simulink model "umich_2d_walking"  (R2012b)
settings: Solver=ode3  StartTime=0.0  StopTime=inf  FixedStep=sample_time  RelTol=1e-3
values from neighbouring files (symbols this model uses):
  fcut_unwrap = 50    [init_umich_2d_walking.m]
  fcut_velocity = 100    [init_umich_2d_walking.m]
  sample_time = 1/update_freq    (= 0.001)    [init_umich_2d_walking.m]
undefined symbols (not defined in the file or in its folder): BOOM_MAX_ENCODER_TICKS, boom_mount_angle, BOOM_PITCH_CAL_VALUE_RAD, BOOM_PITCH_CAL_VALUE_TICKS, BOOM_PITCH_ENCODER_RAD_PER_TICK, BOOM_ROLL_CAL_VALUE_RAD, BOOM_ROLL_CAL_VALUE_TICKS, BOOM_ROLL_ENCODER_RAD_PER_TICK, BOOM_YAW_ENCODER_RAD_PER_TICK, control_start_time, desired_torso_pitch, DiscIntNeverNeededParam, fcut_acceleration, gd, get, h_alpha, HIP_ABS_ENCODER_RAD_PER_TICK, hip_gravity_compensation, HIP_INC_ENCODER_RAD_PER_TICK, HIP_INC_MAX_ENCODER_TICKS, HIP_MOTOR_CONSTANT, HIP_MTR_GEAR_RATIO, HIP_MTR_MAX_TORQUE, i_limit_lateral, j_motor_reflected, k_leg_spring, kd_lateral, kd_pitch, kd_sea_torque, ki_lateral, kp_lateral, kp_pitch, kp_sea_torque, lateral_torque_ramp_time, LEFT_HIP_CALIB_POS, LEFT_HIP_CALIB_VAL, LEFT_MOTOR_HIP_DIRECTION, LEG1_LEG_A_CALIB_VAL, LEG1_LEG_A_RAD_PER_CNT, LEG1_LEG_B_CALIB_VAL, LEG1_LEG_B_RAD_PER_CNT, LEG1_MOTOR_A_DIRECTION, LEG1_MOTOR_B_DIRECTION, LEG1_TRAN_A_CALIB_VAL, LEG1_TRAN_A_RAD_PER_CNT, LEG1_TRAN_B_CALIB_VAL, LEG1_TRAN_B_RAD_PER_CNT, LEG2_LEG_A_CALIB_VAL, LEG2_LEG_A_RAD_PER_CNT, LEG2_LEG_B_CALIB_VAL, LEG2_LEG_B_RAD_PER_CNT, LEG2_MOTOR_A_DIRECTION, LEG2_MOTOR_B_DIRECTION, LEG2_TRAN_A_CALIB_VAL, LEG2_TRAN_A_RAD_PER_CNT, LEG2_TRAN_B_CALIB_VAL, LEG2_TRAN_B_RAD_PER_CNT, LEG_A_CALIB_LOC, LEG_B_CALIB_LOC, LEG_MOTOR_CONSTANT ... (+23)
libraries: xpcethercatlib x160, simulink x9, dspswit3 x1
(part 3 of 3)

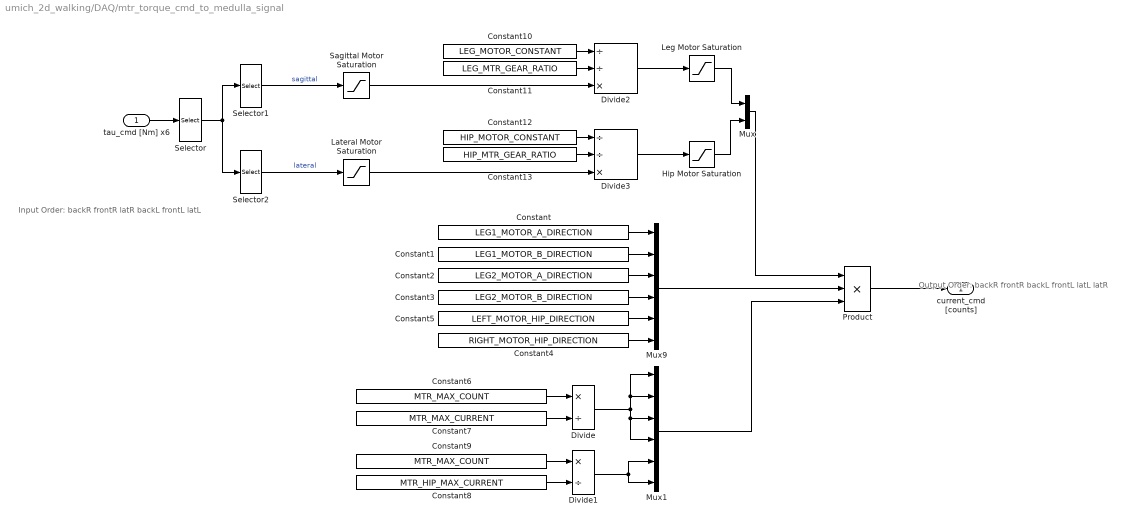
== system umich_2d_walking/DAQ/mtr_torque_cmd_to_medulla_signal ==
  note: Input Order:
      |
      | backR
      | frontR
      | latR
      | backL
      | frontL
      | latL
  note: Output Order:
      |
      | backR
      | frontR
      | backL
      | frontL
      | latL
      | latR
  tau_cmd [Nm] x6 : Inport
  " Lateral Motor Saturation" : Saturate  UpperLimit=HIP_MTR_MAX_TORQUE  LowerLimit=-HIP_MTR_MAX_TORQUE
      settings: AttributesFormatString=Top: %<UpperLimit>\nBottom: %<LowerLimit>
  " Sagittal Motor Saturation" : Saturate  UpperLimit=LEG_MTR_MAX_TORQUE  LowerLimit=-LEG_MTR_MAX_TORQUE
      settings: AttributesFormatString=Top: %<UpperLimit>\nBottom: %<LowerLimit>
  Constant : Constant  Value=LEG1_MOTOR_A_DIRECTION
  Constant1 : Constant  Value=LEG1_MOTOR_B_DIRECTION
  Constant10 : Constant  Value=LEG_MOTOR_CONSTANT
  Constant11 : Constant  Value=LEG_MTR_GEAR_RATIO
  Constant12 : Constant  Value=HIP_MOTOR_CONSTANT
  Constant13 : Constant  Value=HIP_MTR_GEAR_RATIO
  Constant2 : Constant  Value=LEG2_MOTOR_A_DIRECTION
  Constant3 : Constant  Value=LEG2_MOTOR_B_DIRECTION
  Constant4 : Constant  Value=RIGHT_MOTOR_HIP_DIRECTION
  Constant5 : Constant  Value=LEFT_MOTOR_HIP_DIRECTION
  Constant6 : Constant  Value=MTR_MAX_COUNT
  Constant7 : Constant  Value=MTR_MAX_CURRENT
  Constant8 : Constant  Value=MTR_HIP_MAX_CURRENT
  Constant9 : Constant  Value=MTR_MAX_COUNT
  Divide : Product  Inputs=*/
  Divide1 : Product  Inputs=*/
  Divide2 : Product  Inputs=//*
  Divide3 : Product  Inputs=//*
  Hip Motor Saturation : Saturate  UpperLimit=10  LowerLimit=-10
      settings: AttributesFormatString=Top: %<UpperLimit>\nBottom: %<LowerLimit>
  Leg Motor Saturation : Saturate  UpperLimit=30  LowerLimit=-30
      settings: AttributesFormatString=Top: %<UpperLimit>\nBottom: %<LowerLimit>
  Mux : Mux  Inputs=2
  Mux1 : Mux  Inputs=6
  Mux9 : Mux  Inputs=6
  Product : Product  Inputs=3  RndMeth=Zero
  Selector : Selector  InputPortWidth=6  IndexOptions=Index vector (dialog)  Indices=[1 2 4 5 6 3]  OutputSizes=1
  Selector1 : Selector  InputPortWidth=6  IndexOptions=Index vector (dialog)  Indices=[1 2 3 4]  OutputSizes=1
  Selector2 : Selector  InputPortWidth=6  IndexOptions=Index vector (dialog)  Indices=[5 6]  OutputSizes=1
  current_cmd [counts] : Outport
  wires:
  Selector/1 -> Selector2/1, Selector1/1
  tau_cmd [Nm] x6/1 -> Selector/1
  Mux1/1 -> Product/3
  Divide1/1 -> Mux1/5, Mux1/6
  Constant8/1 -> Divide1/2
  Constant9/1 -> Divide1/1
  Divide/1 -> Mux1/1, Mux1/2, Mux1/3, Mux1/4
  Constant7/1 -> Divide/2
  Constant6/1 -> Divide/1
  Product/1 -> current_cmd [counts]/1
  Constant4/1 -> Mux9/6
  Constant5/1 -> Mux9/5
  Constant3/1 -> Mux9/4
  Mux9/1 -> Product/2
  Constant2/1 -> Mux9/3
  Constant1/1 -> Mux9/2
  Constant/1 -> Mux9/1
  Selector1/1 -> " Sagittal Motor Saturation"/1  "sagittal"
  Selector2/1 -> " Lateral Motor Saturation"/1  "lateral"
  Constant11/1 -> Divide2/2
  Constant10/1 -> Divide2/1
  Constant13/1 -> Divide3/2
  Constant12/1 -> Divide3/1
  Divide3/1 -> Hip Motor Saturation/1
  Divide2/1 -> Leg Motor Saturation/1
  Mux/1 -> Product/1
  Leg Motor Saturation/1 -> Mux/1
  Hip Motor Saturation/1 -> Mux/2
  " Sagittal Motor Saturation"/1 -> Divide2/3
  " Lateral Motor Saturation"/1 -> Divide3/3

== system umich_2d_walking/DAQ/unwrap_encoders ==
  Encoder Readings : Inport
  Demux : Demux  Outputs=3
  Mux : Mux
  Selector : Selector  InputPortWidth=15  IndexOptions=Index vector (dialog)  Indices=[10 12 14]  OutputSizes=1
  Selector1 : Selector  InputPortWidth=18  IndexOptions=Index vector (dialog)  Indices=[1 2 3 4 5 6 7 8 9 16 11 17 13 18 15]  OutputSizes=1
  unwrap_boom_yaw_encoder : Subsystem
  unwrap_lateral_incremental_encoders Left : Subsystem
  unwrap_lateral_incremental_encoders Right : Subsystem
  Adjusted Encoder Readings : Outport
  wires:
  Mux/1 -> Selector1/1
  Selector1/1 -> Adjusted Encoder Readings/1
  unwrap_boom_yaw_encoder/1(continuous [ticks]) -> Mux/4
  unwrap_lateral_incremental_encoders Right/1(continuous [ticks]) -> Mux/3
  unwrap_lateral_incremental_encoders Left/1(continuous [ticks]) -> Mux/2
  Demux/3 -> unwrap_boom_yaw_encoder/1(wrapped [ticks])
  Demux/2 -> unwrap_lateral_incremental_encoders Right/1(wrapped [ticks])
  Demux/1 -> unwrap_lateral_incremental_encoders Left/1(wrapped [ticks])
  Selector/1 -> Demux/1
  Encoder Readings/1 -> Selector/1, Mux/1

== system umich_2d_walking/UMich Controller/Opposing Pulses ==
  Gain : Gain  Gain=-1
  Gain1 : Gain  Gain=-1
  Mux1 : Mux  Inputs=6
  Sum1 : Sum  Inputs=|++
  neg_tau : DiscretePulseGenerator  PulseType=Time based  Amplitude=-4.8  PulseWidth=10  PhaseDelay=1
  pos_tau : DiscretePulseGenerator  PulseType=Time based  Amplitude=4.8  PulseWidth=10
  u : Outport
  wires:
  Gain1/1 -> Mux1/4
  Sum1/1 -> Mux1/1, Gain/1, Mux1/3, Gain1/1, Mux1/5, Mux1/6
  Mux1/1 -> u/1
  pos_tau/1 -> Sum1/1
  Gain/1 -> Mux1/2
  neg_tau/1 -> Sum1/2

== system umich_2d_walking/UMich Controller/Torso Pitch Control ==
  q_um : Inport
  dq_um : Inport  Port=2
  Proportional Gain1 : Gain  Description=xPCTag(1)=kp_pitch;  Gain=kp_pitch
  Proportional Gain2 : Gain  Description=xPCTag(1)=kd_pitch;  Gain=kd_pitch
  Saturation : Saturate  UpperLimit=25*pi/180  LowerLimit=-25*pi/180
  Selector2 : Selector  InputPortWidth=13  IndexOptions=Index vector (dialog)  Indices=[3]  OutputSizes=1
  Selector5 : Selector  InputPortWidth=13  IndexOptions=Index vector (dialog)  Indices=[3]  OutputSizes=1
  Sum1 : Sum  Inputs=|+-
  Sum2 : Sum  Inputs=++|
  Sum3 : Sum  Inputs=|+-
  Sum4 : Sum  Inputs=|++
  desired_pitch : Constant  Value=desired_torso_pitch
  desired_pitch_velocity : Constant  Value=0
  torso_pitch_offset : Constant  Value=desired_torso_pitch
  out : Outport
  wires:
  q_um/1 -> Selector5/1
  desired_pitch/1 -> Sum1/1
  Sum1/1 -> Proportional Gain1/1
  Saturation/1 -> out/1
  torso_pitch_offset/1 -> Sum2/1
  Selector2/1 -> Sum3/2
  dq_um/1 -> Selector2/1
  Selector5/1 -> Sum1/2
  desired_pitch_velocity/1 -> Sum3/1
  Sum3/1 -> Proportional Gain2/1
  Sum4/1 -> Sum2/2
  Proportional Gain2/1 -> Sum4/2
  Proportional Gain1/1 -> Sum4/1
  Sum2/1 -> Saturation/1

== system umich_2d_walking/UMich Controller/Zero ==
  Mux1 : Mux  Inputs=6
  zero : Constant  Value=0
  u : Outport
  wires:
  Mux1/1 -> u/1
  zero/1 -> Mux1/1, Mux1/2, Mux1/3, Mux1/4, Mux1/5, Mux1/6

== system umich_2d_walking/UMich Controller/cmu_to_um ==
  note: UMich Order:
      |
      | boomYaw
      | boomRoll
      | boomPitch
      |
      | backJointR
      | frontJointR
      | backGearR
      | frontGearR
      | latR
      |
      | backJointL
      | frontJointL
      | backGearL
      | frontGearL
      | latL
  note: CMU Order:
      |
      | backJointR
      | backGearR
      | frontJointR
      | frontGearR
      |
      | backJointL
      | backGearL
      | frontJointL
      | frontGearL
      |
      | latR
      | latL
      |
      | boomRoll
      | boomYaw
      | boomPitch
  q_cmu : Inport
  dq_cmu : Inport  Port=2
  Constant2 : Constant  Value=2*pi
  Gain : Gain  Gain=-1
  Gain1 : Gain  Gain=-1
  Gain2 : Gain  Gain=-1
  Mux1 : Mux  Inputs=3
  Mux3 : Mux  Inputs=3
  Selector : Selector  InputPortWidth=13  IndexOptions=Index vector (dialog)  Indices=[1 2 3 4 5 6 7 8]  OutputSizes=1
  Selector1 : Selector  InputPortWidth=13  IndexOptions=Index vector (dialog)  Indices=[9 10 11 12]  OutputSizes=1
  Selector2 : Selector  InputPortWidth=13  IndexOptions=Index vector (dialog)  Indices=[1 2 3 4 5 6 7 8]  OutputSizes=1
  Selector3 : Selector  InputPortWidth=13  IndexOptions=Index vector (dialog)  Indices=[9 10 11 12]  OutputSizes=1
  Selector4 : Selector  InputPortWidth=13  IndexOptions=Index vector (dialog)  Indices=[13]  OutputSizes=1
  Selector5 : Selector  InputPortWidth=13  IndexOptions=Index vector (dialog)  Indices=[13]  OutputSizes=1
  Sum2 : Sum  Inputs=+-|
  dq_cmu_to_um_order : Selector  InputPortWidth=13  IndexOptions=Index vector (dialog)  Indices=[12 11 13 1 3 2 4 9 5 7 6 8 10]  OutputSizes=1
  q_cmu_to_um_order : Selector  InputPortWidth=13  IndexOptions=Index vector (dialog)  Indices=[12 11 13 1 3 2 4 9 5 7 6 8 10]  OutputSizes=1
  q_um : Outport
  dq_um : Outport  Port=2
  wires:
  q_cmu_to_um_order/1 -> q_um/1
  Constant2/1 -> Sum2/1
  Mux3/1 -> q_cmu_to_um_order/1
  Sum2/1 -> Mux3/1
  Selector/1 -> Sum2/2
  q_cmu/1 -> Selector/1, Selector5/1, Selector1/1
  Selector1/1 -> Mux3/2
  dq_cmu/1 -> Selector4/1, Selector3/1, Selector2/1
  Selector3/1 -> Mux1/2
  Selector2/1 -> Gain/1
  Gain/1 -> Mux1/1
  Mux1/1 -> dq_cmu_to_um_order/1
  dq_cmu_to_um_order/1 -> dq_um/1
  Selector4/1 -> Gain2/1
  Selector5/1 -> Gain1/1
  Gain1/1 -> Mux3/3
  Gain2/1 -> Mux1/3

== system umich_2d_walking/UMich Controller/lateral_PID_control ==
  q_cmu : Inport
  dq_cmu : Inport  Port=2
  Demux1 : Demux  Outputs=2
  Gain : Gain  Gain=-1
  Gain1 : Gain  Gain=-1
  Lateral Hip PID : Subsystem
  Motor Saturation : Saturate  UpperLimit=max_torque_lateral  LowerLimit=-max_torque_lateral
      settings: AttributesFormatString=Top: %<UpperLimit>\nBottom: %<LowerLimit>
  Mux : Mux  Inputs=2
  Mux1 : Mux  Inputs=2
  Sum1 : Sum  Inputs=|+-
  Sum2 : Sum  Inputs=|+-
  Sum4 : Sum  Inputs=++|
  desired_velocity : Constant  Value=0
  feedforward_torque (gravity compensation) : Constant  Value=hip_gravity_compensation
  select_dqLateral : Selector  InputPortWidth=13  IndexOptions=Index vector (dialog)  Indices=[9 10]  OutputSizes=1
  select_qLateral : Selector  InputPortWidth=13  IndexOptions=Index vector (dialog)  Indices=[9 10]  OutputSizes=1
  spherical_correction_angle : Subsystem
  tau_lateral : Outport
  wires:
  spherical_correction_angle/1(lateral_correction [rad]) -> Mux/1, Gain/1
  Lateral Hip PID/1(out) -> Sum4/2
  Sum2/1 -> Lateral Hip PID/1(position_error)
  q_cmu/1 -> spherical_correction_angle/1(q_cmu), select_qLateral/1
  select_dqLateral/1 -> Sum1/2
  dq_cmu/1 -> select_dqLateral/1
  Mux1/1 -> Motor Saturation/1
  Demux1/1 -> Gain1/1
  Gain1/1 -> Mux1/1
  Demux1/2 -> Mux1/2
  desired_velocity/1 -> Sum1/1
  Sum1/1 -> Lateral Hip PID/2(velocity_error)
  Sum4/1 -> Demux1/1
  feedforward_torque (gravity compensation)/1 -> Sum4/1
  Gain/1 -> Mux/2
  Mux/1 -> Sum2/1
  select_qLateral/1 -> Sum2/2  "qLateral"
  Motor Saturation/1 -> tau_lateral/1

== system umich_2d_walking/UMich Controller/tau_um_to_cmu ==
  tau_um : Inport
  Gain : Gain  Gain=-1
  Mux2 : Mux  Inputs=2
  Selector : Selector  InputPortWidth=6  IndexOptions=Index vector (dialog)  Indices=[1 2 3 4 5]  OutputSizes=1
  Selector2 : Selector  InputPortWidth=6  IndexOptions=Index vector (dialog)  Indices=[6]  OutputSizes=1
  tau_cmu : Outport
  wires:
  tau_um/1 -> Selector2/1, Selector/1
  Selector/1 -> Gain/1
  Gain/1 -> Mux2/1
  Mux2/1 -> tau_cmu/1
  Selector2/1 -> Mux2/2

== system umich_2d_walking/Actuator Control/SEA Controller (Position)/filtered_derivative ==
  x : Inport
  Gain1 : Gain  Gain=1/sample_time
  difference : simulink/Discrete/Difference  ICPrevInput=0.0  InputProcessing=Inherited  OutMin=[]  OutMax=[]  OutDataType=fixdt(1, 16)  OutScaling=2^-10  DoSatur=off
  single_pole_filter : DiscreteTransferFcn  Numerator=[(1-exp(-2*pi*fcut_acceleration*sample_time)) 0]  Denominator=[1 -exp(-2*pi*fcut_acceleration*sample_time)]  SampleTime=sample_time
  dx/dt : Outport
  wires:
  Gain1/1 -> difference/1
  difference/1 -> single_pole_filter/1
  x/1 -> Gain1/1
  single_pole_filter/1 -> dx/dt/1

== system umich_2d_walking/DAQ/calibrate_and_convert_to_rad/calibrate_abs_encoder ==
  encoder_ticks : Inport
  cal_pt_ticks : Inport  Port=2
  cal_pt_rad : Inport  Port=3
  ticks_to_rad_const : Inport  Port=4
  Product : Product  RndMeth=Zero
  Sum : Sum  Inputs=|+-
  Sum1 : Sum  Inputs=|++
  angle [rad] : Outport
  wires:
  Sum/1 -> Product/1  "tick_diff"
  encoder_ticks/1 -> Sum/1  "encoder_ticks"
  Product/1 -> Sum1/1  "rad_diff"
  ticks_to_rad_const/1 -> Product/2  "ticks_to_rad_const"
  cal_pt_ticks/1 -> Sum/2  "calibration_point_ticks"
  Sum1/1 -> angle [rad]/1  "calibrated_angle"
  cal_pt_rad/1 -> Sum1/2  "calibration_point_radians"

== system umich_2d_walking/DAQ/calibrate_and_convert_to_rad/calibration_pt_radians ==
  Constant{1,3,5,7} (4 alike) : Constant  Value=LEG_A_CALIB_LOC
  Constant10 : Constant  Value=LEFT_HIP_CALIB_POS
  Constant11 : Constant  Value=BOOM_ROLL_CAL_VALUE_RAD
  Constant12 : Constant  Value=BOOM_PITCH_CAL_VALUE_RAD
  Constant{2,4,6,8} (4 alike) : Constant  Value=LEG_B_CALIB_LOC
  Constant9 : Constant  Value=RIGHT_HIP_CALIB_POS
  Mux3 : Mux  Inputs=12
  calibration_pt [rad] : Outport
  wires:
  Constant4/1 -> Mux3/4
  Constant8/1 -> Mux3/8
  Constant3/1 -> Mux3/1
  Mux3/1 -> calibration_pt [rad]/1
  Constant11/1 -> Mux3/11
  Constant6/1 -> Mux3/7
  Constant12/1 -> Mux3/12
  Constant9/1 -> Mux3/10
  Constant2/1 -> Mux3/3
  Constant5/1 -> Mux3/6
  Constant1/1 -> Mux3/2
  Constant10/1 -> Mux3/9
  Constant7/1 -> Mux3/5

== system umich_2d_walking/DAQ/calibrate_and_convert_to_rad/calibration_pt_ticks ==
  Constant1 : Constant  Value=LEG2_TRAN_A_CALIB_VAL
  Constant10 : Constant  Value=LEFT_HIP_CALIB_VAL
  Constant11 : Constant  Value=BOOM_ROLL_CAL_VALUE_TICKS
  Constant12 : Constant  Value=BOOM_PITCH_CAL_VALUE_TICKS
  Constant2 : Constant  Value=LEG2_LEG_B_CALIB_VAL
  Constant3 : Constant  Value=LEG2_LEG_A_CALIB_VAL
  Constant4 : Constant  Value=LEG2_TRAN_B_CALIB_VAL
  Constant5 : Constant  Value=LEG1_TRAN_A_CALIB_VAL
  Constant6 : Constant  Value=LEG1_LEG_B_CALIB_VAL
  Constant7 : Constant  Value=LEG1_LEG_A_CALIB_VAL
  Constant8 : Constant  Value=LEG1_TRAN_B_CALIB_VAL
  Constant9 : Constant  Value=RIGHT_HIP_CALIB_VAL
  Mux3 : Mux  Inputs=12
  calibration_pt [ticks] : Outport
  wires:
  Constant3/1 -> Mux3/5
  Constant10/1 -> Mux3/9
  Constant5/1 -> Mux3/2
  Constant1/1 -> Mux3/6
  Constant6/1 -> Mux3/3
  Constant9/1 -> Mux3/10
  Constant12/1 -> Mux3/12
  Constant2/1 -> Mux3/7
  Constant11/1 -> Mux3/11
  Mux3/1 -> calibration_pt [ticks]/1
  Constant7/1 -> Mux3/1
  Constant4/1 -> Mux3/8
  Constant8/1 -> Mux3/4

== system umich_2d_walking/DAQ/calibrate_and_convert_to_rad/ticks_to_radians_constants ==
  Constant1 : Constant  Value=LEG2_TRAN_A_RAD_PER_CNT
  Constant10 : Constant  Value=-HIP_ABS_ENCODER_RAD_PER_TICK
  Constant11 : Constant  Value=BOOM_ROLL_ENCODER_RAD_PER_TICK
  Constant12 : Constant  Value=BOOM_PITCH_ENCODER_RAD_PER_TICK
  Constant2 : Constant  Value=LEG2_LEG_B_RAD_PER_CNT
  Constant3 : Constant  Value=LEG2_LEG_A_RAD_PER_CNT
  Constant4 : Constant  Value=LEG2_TRAN_B_RAD_PER_CNT
  Constant5 : Constant  Value=LEG1_TRAN_A_RAD_PER_CNT
  Constant6 : Constant  Value=LEG1_LEG_B_RAD_PER_CNT
  Constant7 : Constant  Value=LEG1_LEG_A_RAD_PER_CNT
  Constant8 : Constant  Value=LEG1_TRAN_B_RAD_PER_CNT
  Constant9 : Constant  Value=HIP_ABS_ENCODER_RAD_PER_TICK
  Mux3 : Mux  Inputs=12
  ticks_to_rad_constants : Outport
  wires:
  Constant3/1 -> Mux3/5
  Constant9/1 -> Mux3/9
  Constant5/1 -> Mux3/2
  Constant1/1 -> Mux3/6
  Constant6/1 -> Mux3/3
  Constant10/1 -> Mux3/10
  Constant12/1 -> Mux3/12
  Constant2/1 -> Mux3/7
  Constant11/1 -> Mux3/11
  Mux3/1 -> ticks_to_rad_constants/1
  Constant7/1 -> Mux3/1
  Constant4/1 -> Mux3/8
  Constant8/1 -> Mux3/4

== system umich_2d_walking/DAQ/hold_initial_lateral_angles/Initial Lateral Hip Angles [rad] ==
  In : Inport
  Enable : EnablePort  StatesWhenEnabling=reset
  Out : Outport
  wires:
  In/1 -> Out/1

== system umich_2d_walking/DAQ/unwrap_encoders/unwrap_boom_yaw_encoder ==
  note: Recommended if-then structure for assigning
      | constants. The criterion '~=0' is realized as cpu register
      | shift when compiling.  The resulting code is fast.
  note: Transform Wrapped Angle into Continuous Angle
  note: predicted angle:
      | phi' = phi_(n-1) + dphi
      | = phi_(n-1) + phi_(n-1)-phi_(n-2)
  wrapped [ticks] : Inport
  1/BOOM_MAX_ENCODER_TICKS : Gain  Gain=1/BOOM_MAX_ENCODER_TICKS
  Abs : Abs
  BOOM_MAX_ENCODER_TICKS : Gain  Gain=BOOM_MAX_ENCODER_TICKS
  Compare To Zero : simulink/Logic and Bit Operations/Compare To Zero  relop=>  OutDataTypeStr=uint8
  Discrete Single Pole Lowpass Filter : DiscreteTransferFcn  Numerator=[(1-exp(-2*pi*fcut_unwrap*sample_time)) 0]  Denominator=[1 -exp(-2*pi*fcut_unwrap*sample_time)]  SampleTime=sample_time
  Gain2 : Gain  Gain=2
  Product : Product  RndMeth=Zero
  Rounding Function : Rounding
  Sum : Sum  Inputs=|+-
  Sum1 : Sum  Inputs=|++
  Sum2 : Sum  Inputs=|++
  Sum3 : Sum  Inputs=-+|
  Switch : Switch  Criteria=u2 ~= 0
      settings: AttributesFormatString=%<Criteria>
  Unit Delay phi_(n-1) : UnitDelay  SampleTime=-1
      settings: AttributesFormatString=initial condition = %<X0>
  Unit Delay phi_(n-2) : UnitDelay  SampleTime=-1
      settings: AttributesFormatString=initial condition = %<X0>
  const : Constant  Value=0.5
  no : Constant  Value=-1
  yes : Constant
  continuous [ticks] : Outport
  wires:
  Discrete Single Pole Lowpass Filter/1 -> Unit Delay phi_(n-1)/1
  Compare To Zero/1 -> Switch/2
  Unit Delay phi_(n-2)/1 -> Sum/2
  yes/1 -> Switch/1
  no/1 -> Switch/3
  Switch/1 -> Product/2
  Rounding Function/1 -> BOOM_MAX_ENCODER_TICKS/1
  wrapped [ticks]/1 -> Sum1/1, Sum3/1
  Product/1 -> Sum1/2
  Abs/1 -> 1/BOOM_MAX_ENCODER_TICKS/1
  1/BOOM_MAX_ENCODER_TICKS/1 -> Sum2/1
  const/1 -> Sum2/2
  Sum2/1 -> Rounding Function/1
  Sum1/1 -> continuous [ticks]/1, Discrete Single Pole Lowpass Filter/1
  BOOM_MAX_ENCODER_TICKS/1 -> Product/1
  Unit Delay phi_(n-1)/1 -> Unit Delay phi_(n-2)/1, Gain2/1
  Gain2/1 -> Sum/1
  Sum/1 -> Sum3/2
  Sum3/1 -> Abs/1, Compare To Zero/1  "phi'-phi"

== system umich_2d_walking/DAQ/unwrap_encoders/unwrap_lateral_incremental_encoders Left ==
  note: Recommended if-then structure for assigning
      | constants. The criterion '~=0' is realized as cpu register
      | shift when compiling.  The resulting code is fast.
  note: Transform Wrapped Angle into Continuous Angle
  note: predicted angle:
      | phi' = phi_(n-1) + dphi
      | = phi_(n-1) + phi_(n-1)-phi_(n-2)
  wrapped [ticks] : Inport
  1/HIP_INC_MAX_ENCODER_TICKS : Gain  Gain=1/HIP_INC_MAX_ENCODER_TICKS
  Abs : Abs
  Compare To Zero : simulink/Logic and Bit Operations/Compare To Zero  relop=>  OutDataTypeStr=uint8
  Discrete Single Pole Lowpass Filter : DiscreteTransferFcn  Numerator=[(1-exp(-2*pi*fcut_unwrap*sample_time)) 0]  Denominator=[1 -exp(-2*pi*fcut_unwrap*sample_time)]  SampleTime=sample_time
  Gain2 : Gain  Gain=2
  HIP_INC_MAX_ENCODER_TICKS : Gain  Gain=HIP_INC_MAX_ENCODER_TICKS
  Product : Product  RndMeth=Zero
  Rounding Function : Rounding
  Sum : Sum  Inputs=|+-
  Sum1 : Sum  Inputs=|++
  Sum2 : Sum  Inputs=|++
  Sum3 : Sum  Inputs=-+|
  Switch : Switch  Criteria=u2 ~= 0
      settings: AttributesFormatString=%<Criteria>
  Unit Delay phi_(n-1) : UnitDelay  SampleTime=-1
      settings: AttributesFormatString=initial condition = %<X0>
  Unit Delay phi_(n-2) : UnitDelay  SampleTime=-1
      settings: AttributesFormatString=initial condition = %<X0>
  const : Constant  Value=0.5
  no : Constant  Value=-1
  yes : Constant
  continuous [ticks] : Outport
  wires:
  Discrete Single Pole Lowpass Filter/1 -> Unit Delay phi_(n-1)/1
  Compare To Zero/1 -> Switch/2
  Unit Delay phi_(n-2)/1 -> Sum/2
  yes/1 -> Switch/1
  no/1 -> Switch/3
  Switch/1 -> Product/2
  Rounding Function/1 -> HIP_INC_MAX_ENCODER_TICKS/1
  wrapped [ticks]/1 -> Sum1/1, Sum3/1
  Product/1 -> Sum1/2
  Abs/1 -> 1/HIP_INC_MAX_ENCODER_TICKS/1
  1/HIP_INC_MAX_ENCODER_TICKS/1 -> Sum2/1
  const/1 -> Sum2/2
  Sum2/1 -> Rounding Function/1
  Sum1/1 -> Discrete Single Pole Lowpass Filter/1, continuous [ticks]/1
  HIP_INC_MAX_ENCODER_TICKS/1 -> Product/1
  Unit Delay phi_(n-1)/1 -> Unit Delay phi_(n-2)/1, Gain2/1
  Gain2/1 -> Sum/1
  Sum/1 -> Sum3/2
  Sum3/1 -> Abs/1, Compare To Zero/1  "phi'-phi"

== system umich_2d_walking/DAQ/unwrap_encoders/unwrap_lateral_incremental_encoders Right ==
  note: predicted angle:
      | phi' = phi_(n-1) + dphi
      | = phi_(n-1) + phi_(n-1)-phi_(n-2)
  note: Transform Wrapped Angle into Continuous Angle
  note: Recommended if-then structure for assigning
      | constants. The criterion '~=0' is realized as cpu register
      | shift when compiling.  The resulting code is fast.
  wrapped [ticks] : Inport
  1/HIP_INC_MAX_ENCODER_TICKS : Gain  Gain=1/HIP_INC_MAX_ENCODER_TICKS
  Abs : Abs
  Compare To Zero : simulink/Logic and Bit Operations/Compare To Zero  relop=>  OutDataTypeStr=uint8
  Discrete Single Pole Lowpass Filter : DiscreteTransferFcn  Numerator=[(1-exp(-2*pi*fcut_unwrap*sample_time)) 0]  Denominator=[1 -exp(-2*pi*fcut_unwrap*sample_time)]  SampleTime=sample_time
  Gain2 : Gain  Gain=2
  HIP_INC_MAX_ENCODER_TICKS : Gain  Gain=HIP_INC_MAX_ENCODER_TICKS
  Product : Product  RndMeth=Zero
  Rounding Function : Rounding
  Sum : Sum  Inputs=|+-
  Sum1 : Sum  Inputs=|++
  Sum2 : Sum  Inputs=|++
  Sum3 : Sum  Inputs=-+|
  Switch : Switch  Criteria=u2 ~= 0
      settings: AttributesFormatString=%<Criteria>
  Unit Delay phi_(n-1) : UnitDelay  SampleTime=-1
      settings: AttributesFormatString=initial condition = %<X0>
  Unit Delay phi_(n-2) : UnitDelay  SampleTime=-1
      settings: AttributesFormatString=initial condition = %<X0>
  const : Constant  Value=0.5
  no : Constant  Value=-1
  yes : Constant
  continuous [ticks] : Outport
  wires:
  Sum3/1 -> Compare To Zero/1, Abs/1  "phi'-phi"
  Sum/1 -> Sum3/2
  Gain2/1 -> Sum/1
  Unit Delay phi_(n-1)/1 -> Gain2/1, Unit Delay phi_(n-2)/1
  HIP_INC_MAX_ENCODER_TICKS/1 -> Product/1
  Sum1/1 -> continuous [ticks]/1, Discrete Single Pole Lowpass Filter/1
  Sum2/1 -> Rounding Function/1
  const/1 -> Sum2/2
  1/HIP_INC_MAX_ENCODER_TICKS/1 -> Sum2/1
  Abs/1 -> 1/HIP_INC_MAX_ENCODER_TICKS/1
  Product/1 -> Sum1/2
  wrapped [ticks]/1 -> Sum3/1, Sum1/1
  Rounding Function/1 -> HIP_INC_MAX_ENCODER_TICKS/1
  Switch/1 -> Product/2
  no/1 -> Switch/3
  yes/1 -> Switch/1
  Unit Delay phi_(n-2)/1 -> Sum/2
  Compare To Zero/1 -> Switch/2
  Discrete Single Pole Lowpass Filter/1 -> Unit Delay phi_(n-1)/1

== system umich_2d_walking/UMich Controller/lateral_PID_control/Lateral Hip PID ==
  position_error : Inport
  velocity_error : Inport  Port=2
  Discrete-Time Integrator : DiscreteIntegrator  IntegratorMethod=Integration: Trapezoidal  SampleTime=sample_time  LimitOutput=on  UpperSaturationLimit=i_limit_lateral  LowerSaturationLimit=-i_limit_lateral  ICPrevOutput=DiscIntNeverNeededParam  ICPrevScaledInput=DiscIntNeverNeededParam
  Proportional Gain : Gain  Description=xPCTag(1)=kp_lateral;  Gain=kp_lateral
  Proportional Gain1 : Gain  Description=xPCTag(1)=kd_lateral;  Gain=kd_lateral
  Proportional Gain2 : Gain  Description=xPCTag(1)=ki_lateral;  Gain=ki_lateral
  Sum : Sum  Inputs=+++
  out : Outport
  wires:
  velocity_error/1 -> Proportional Gain1/1
  Discrete-Time Integrator/1 -> Sum/3
  Proportional Gain2/1 -> Discrete-Time Integrator/1
  Proportional Gain/1 -> Sum/2
  position_error/1 -> Proportional Gain2/1, Proportional Gain/1
  Sum/1 -> out/1
  Proportional Gain1/1 -> Sum/1

== system umich_2d_walking/UMich Controller/lateral_PID_control/spherical_correction_angle ==
  q_cmu : Inport
  Selector : Selector  InputPortWidth=13  IndexOptions=Index vector (dialog)  Indices=[11]  OutputSizes=1
  Sum1 : Sum  Inputs=|+-
  Terminator2 : Terminator
  boom_mount_angle : Constant  Value=boom_mount_angle
  lateral_correction : Gain  Gain=180/pi
  lateral_correction [rad] : Outport
  wires:
  Sum1/1 -> lateral_correction/1, lateral_correction [rad]/1
  Selector/1 -> Sum1/1  "qBoomRoll"
  q_cmu/1 -> Selector/1
  boom_mount_angle/1 -> Sum1/2
  lateral_correction/1 -> Terminator2/1

== matlab function umich_2d_walking/UMich Controller/controller ==
  data: t input; u output; y output; x input; theta_limits input; dy output; h_alpha input; poly_cor input; kp input; kd input; epsilon input; qTdesired input; pdCtrl input; pdPlusFwdCtrl input; L2fhCtrl input; auto_swap input; swap_cmd input; prev_leg parameter; sat_val input; stance_leg_manual input; scuff input; fix_s input; s_freq input; q3_des input; swap input; swap_threshold input; stance_leg input; s output; ds output; pd output; stance_leg_next output
function [u,y,dy,s,ds,pd,stance_leg_next] = ...
   controller(t,x,theta_limits, h_alpha, poly_cor,kp,kd,epsilon,qTdesired, ...
   pdCtrl,pdPlusFwdCtrl,L2fhCtrl,auto_swap,swap_cmd,prev_leg,...
   sat_val, stance_leg_manual, scuff,fix_s,s_freq,q3_des,swap,swap_threshold, stance_leg)
%%eml


% CMU Notes:
% ----------

% General referemce: 
% Ref1 = Chevallereau et al. 2009. Asymptotically stable walking of 
%        a five-link underactuated 3-d bipedal robot


% Michigan ATRIAS coordinate system:

% q1 = BoomYaw
% q2 = BoomRoll
% q3 = BoomPitch

% q4 = BackJointR 
% q5 = FrontJointR
% q6 = BackGearR
% q7 = FrontGearR
% q8 = LatR

% q9 = BackJointL 
% q10 = FrontJointL
% q11 = BackGearL
% q12 = FrontGearL
% q13 = LatL



% ----------------------------
% Extract 2D Coordinate System
% ----------------------------

% get angles and corresponding velocities
q  = x(1:13);
dq = x(14:26);

% reduce to 2D angles (remove lateral components)
q2d  = q([1:7 9:12]); 
dq2d = dq([1:7 9:12]);

% Resulting 2d coordinate system:

% q2d1 = BoomYaw
% q2d2 = BoomRoll
% q2d3 = BoomPitch

% q2d4 = BackJointR 
% q2d5 = FrontJointR
% q2d6 = BackGearR
% q2d7 = FrontGearR
% q2d8 = BackJointL 
% q2d9 = FrontJointL
% q2d10 = BackGearL
% q2d11 = FrontGearL



% -------------------------------
% Compute Current ATRIAS Dynamics
% -------------------------------

% load estimated robot parameters: masses, lengths, inertias, etc.
% from file 
[g mTotal L1 L2 L3 L4 m1 m2 m3 m4 Jcm1 Jcm2 Jcm3 Jcm4 ellzcm1 ellzcm2 ellzcm3 ellzcm4 ellycm1 ellycm2 ellycm3 ellycm4 LT mT JcmT ellzcmT ellycmT mH JcmH ...
    K1 K2 Kd1 Kd2 Jrotor1 Jrotor2 Jgear1  Jgear2 R1  R2 Kfric_HarmonicDrive] = modelParametersAtrias_v05;

% compute Euler-Lagrange equation components
% D*ddq + C*dq + G = B*u - F_damping_torque
% D = mass matrix
% C = coriolis matrix
% G = gravity vector
% B = input matrix
% DampingSpringTorque = vector of damping torques of the series springs
[D C G B DampingSpringTorque]= LagrangeModelAtriasFlight2D(q2d,dq2d);

% Create B for harmonic drives of ATRIAS 2.1
% note: matrix is 11x4 for four actuated motors
B_HarmonicDrive=zeros(11,4);

% assign motor inputs to matrix assuming
% u = [u1 u2 u3 u4]
% with u1: right back motor
%      u2: right front motor
%      u3: left back motor
%      u4: left front motor
B_HarmonicDrive( 6,1) =1;
B_HarmonicDrive( 7,2) =1; % 
B_HarmonicDrive(10,3) =1;
B_HarmonicDrive(11,4) =1;



% --------------------------------------
% Assign Feedback Control Gain Constants
% --------------------------------------

% note: kp, kd and epsilon provided from GUI
%       kp and kd are 3x1 vectors according to the control of 
%       leg length, leg splay, and lateral position

% proportional gain constants 
kp = kp/epsilon^2;

% derivative gain constants
kd = kd/epsilon;



% --------------------------------------
% Compute Sagittal Plane Control Torques
% --------------------------------------

% note: that is torque inputs u1 to u4 summarized in variable u12

% summarize coriolins, gravity and damping terms in one big matrix H
H = C*dq2d + G + DampingSpringTorque + B_HarmonicDrive*(Kfric_HarmonicDrive*B_HarmonicDrive')*dq2d;
% note currently Kfric_HarmonicDrive is set to zero; thus, the term 
% B_HarmonicDreive*(Kfric_HarmonicDrive*B_HarmonicDrive')*dq2d does not 
% contribute to H 

% compute control torques for sagittal plane
[u12,y12,dy12,s,ds,stance_leg_next,pd] = ...
    ATRIAS2D_SS_feedback_control_RoughGround07(t,q2d,dq2d,D,H,G,B, ...
    theta_limits,h_alpha,poly_cor,kp(1:2),kd(1:2),qTdesired, ...
    pdCtrl,pdPlusFwdCtrl,L2fhCtrl,auto_swap,swap_cmd,...
    stance_leg,scuff,fix_s,s_freq, stance_leg_manual, swap, swap_threshold);



% ----------------------------------------------------------------------        
% Control Lateral PD Control Torques  to Maintain Desired Lateral Angles 
% ----------------------------------------------------------------------

% simple PD control of lateral position
[u3,y3,dy3] = ATRIAS_hip_controller_v2(q, dq, q3_des, kp(3), kd(3));
% note: q3_des is provided from the GUI, just like kp(3) and kd(3)



% ------------------------------------------
% Generate Torque Commands for ATRIAS motors
% ------------------------------------------

% concatenate torque vector according to
% u1 = right back motor
% u2 = right front motor
% u3 = right lateral motor
% u4 = left back motor
% u5 = left front motor
% u6 = left lateral motor
u  = [ u12(1:2);  u3(1);  u12(3:4);  u3(2)];

% concatenate error vector (between desired and current joint positions)
y  = [ y12(1:2);  y3(1);  y12(3:4);  y3(2)];

% concatenate error velocity vecotir
dy = [dy12(1:2); dy3(1); dy12(3:4); dy3(2)];

% set saturation limit vector
sat_val2 = [sat_val(1) sat_val(1) sat_val(2) sat_val(1) sat_val(1) sat_val(2)].';
% note: sat_val is 2x1 vector provided in GUI for sagittal and lateral
% motors

% saturate motor torque commands
u=min(u, sat_val2);
u=max(u,-sat_val2);

end

== matlab function umich_2d_walking/DAQ/Supervisory ==
  data: u input; backLAmp1 output; backLAmp2 output; frontLAmp1 output; frontLAmp2 output; backRAmp1 output; backRAmp2 output; frontRAmp1 output; frontRAmp2 output; backLError output; frontLError output; backRError output; frontRError output; backLMotorV output; backLLogicV output; frontLMotorV output; frontLLogicV output; backRMotorV output; backRLogicV output; frontRMotorV output; frontRLogicV output; frontLTemp0 output; frontLTemp1 output; frontLTemp2 output; frontLTemp3 output; frontLTemp4 output; frontLTemp5 output; backLTemp0 output; backLTemp1 output; backLTemp2 output; backLTemp3 output; backLTemp4 output; backLTemp5 output
function [backLAmp1, backLAmp2, frontLAmp1, frontLAmp2, backRAmp1, ....
    backRAmp2, frontRAmp1, frontRAmp2, backLError, frontLError, ...
    backRError, frontRError, backLMotorV, backLLogicV, frontLMotorV, ...
    frontLLogicV, backRMotorV, backRLogicV, frontRMotorV, frontRLogicV,...
    frontLTemp0, frontLTemp1, frontLTemp2, frontLTemp3, frontLTemp4,...
    frontLTemp5, backLTemp0, backLTemp1, backLTemp2, backLTemp3, ...
    backLTemp4, backLTemp5]    = fcn(u)

 % amplifiers
 backRAmp1 = u(17);
 backRAmp2 = u(18);
 frontRAmp1 = u(37);
 frontRAmp2 = u(38);
 backLAmp1 = u(57);
 backLAmp2 = u(58);
 frontLAmp1 = u(77);
 frontLAmp2 = u(78);
 
 % error flags
 backRError = u(4);
 frontRError = u(24);
 backLError = u(44);
 frontLError = u(64);
 
 % voltages
  backRMotorV = u(9);
  backRLogicV = u(10);
  frontRMotorV = u(29);
  frontRLogicV = u(30);
  backLMotorV = u(49);
  backLLogicV = u(50);
  frontLMotorV = u(69);
  frontLLogicV = u(70);
  
  % temperature
  frontLTemp0 = u(71);
  frontLTemp1 = u(72);
  frontLTemp2 = u(73);
  frontLTemp3 = u(74);
  frontLTemp4 = u(75);
  frontLTemp5 = u(76);
  backLTemp0 = u(51);
  backLTemp1 = u(52);
  backLTemp2 = u(53);
  backLTemp3 = u(54);
  backLTemp4 = u(55);
  backLTemp5 = u(56);
end
